simulink model "pro_simu_obsv"  (R2020b)
settings: Solver=VariableStepAuto  StartTime=0.0  StopTime=6  RelTol=1e-3
values from neighbouring files (symbols this model uses):
  A = subs(Jx,[x1,x2,x3,x4],[0,0,0,0])    [linearisation.m]    (also in pro_main_code.m = [0 1 0 0;0 -15.47 41.68 0;0 0 0 1;0 -14.89 84.05 0])
  B = subs(Ju,u,0)    [linearisation.m]    (also in pro_main_code.m = [0;27.12;0;23.13])
  C = [1 0 0 0]    [pro_main_code.m]
  Gcl0_inv_lqr = inv(Gcl0)    [pro_main_code.m]
  K_11_lqr = K_lqr1(1,1:4)    [pro_main_code.m]
  K_12_lqr = K_lqr1(1,5)    [pro_main_code.m]
  K_lqr = lqr(A,B,QQ,R)    [pro_main_code.m]
  L_lqr = l_lqr'    [pro_main_code.m]
libraries: simulink x1
settings Model: Creator=Benyamin (hamireZ)  LastModifiedBy=Benyamin (hamireZ)

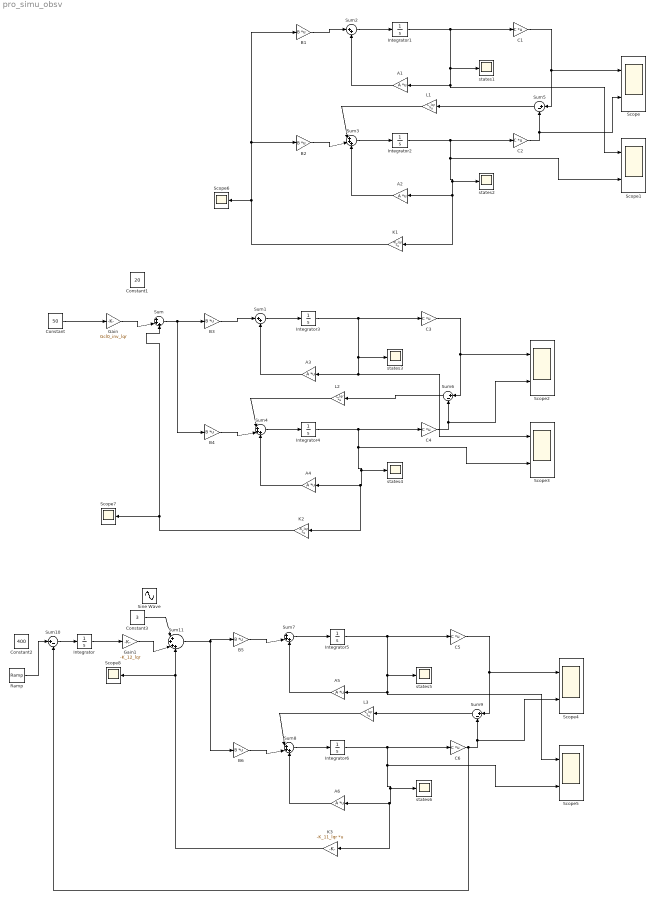
== system pro_simu_obsv ==
  A{1..6} (6 alike) : Gain  Gain=A  Multiplication=Matrix(K*u) (u vector)
  B{1..6} (6 alike) : Gain  Gain=B  Multiplication=Matrix(K*u) (u vector)
  C{1..6} (6 alike) : Gain  Gain=C  Multiplication=Matrix(K*u) (u vector)
  Constant : Constant  Value=50
  Constant1 : Constant  Value=20
  Constant2 : Constant  Value=400
  Constant3 : Constant  Value=3
  Gain : Gain  Gain=Gcl0_inv_lqr
  Gain1 : Gain  Gain=-K_12_lqr
  Integrator : Integrator
  Integrator1 : Integrator  InitialCondition=[1;0;1;0]
  Integrator2 : Integrator  InitialCondition=[-1;0;0;0]
  Integrator3 : Integrator  InitialCondition=[1;1;1;1]
  Integrator4 : Integrator  InitialCondition=[-1;0;-2;-1]
  Integrator5 : Integrator  InitialCondition=[1;1;1;1]
  Integrator6 : Integrator  InitialCondition=[-1;0;-2;-1]
  K1 : Gain  Gain=-K_lqr  Multiplication=Matrix(K*u) (u vector)
  K2 : Gain  Gain=-K_lqr  Multiplication=Matrix(K*u) (u vector)
  K3 : Gain  Gain=-K_11_lqr  Multiplication=Matrix(K*u) (u vector)
  L1 : Gain  Gain=L_lqr  Multiplication=Matrix(K*u) (u vector)
  L2 : Gain  Gain=L_lqr  Multiplication=Matrix(K*u) (u vector)
  L3 : Gain  Gain=L_lqr  Multiplication=Matrix(K*u) (u vector)
  Ramp : simulink/Sources/Ramp  slope=100  start=0  InitialOutput=0
  Scope{,1..5} (6 alike) : Scope  NumInputPorts=2
  Scope6 : Scope
  Scope7 : Scope
  Scope8 : Scope
  Sine Wave : Sin  Frequency=2  SampleTime=0
  Sum{,3..4,7..8} (5 alike) : Sum  Inputs=|+++
  Sum1 : Sum  Inputs=|++
  Sum{5..6,9..10} (4 alike) : Sum  Inputs=|+-
  Sum11 : Sum  Inputs=|++++
  Sum2 : Sum  Inputs=|++
  states{1..6} (6 alike) : Scope
  wires:
  Integrator6/1 -> C6/1, states6/1, A6/1, K3/1, Scope5/2
  B4/1 -> Sum4/2
  Sum1/1 -> Integrator3/1
  Constant/1 -> Gain/1
  Sum10/1 -> Integrator/1
  A3/1 -> Sum1/2
  C5/1 -> Scope4/1, Sum9/1
  Integrator/1 -> Gain1/1
  C4/1 -> Sum6/2, Scope2/2
  Gain1/1 -> Sum11/3
  Sum11/1 -> B5/1, B6/1
  B2/1 -> Sum3/2
  L1/1 -> Sum3/1
  Gain/1 -> Sum/2
  A4/1 -> Sum4/3
  Integrator5/1 -> A5/1, Scope5/1, states5/1, C5/1
  Sum6/1 -> L2/1
  Integrator3/1 -> A3/1, Scope3/1, states3/1, C3/1
  Sum4/1 -> Integrator4/1
  C3/1 -> Scope2/1, Sum6/1
  B5/1 -> Sum7/2
  B6/1 -> Sum8/2
  Integrator1/1 -> C1/1, states1/1, Scope1/1, A1/1
  C6/1 -> Sum9/2, Scope4/2, Sum10/2
  Sum8/1 -> Integrator6/1
  Sum9/1 -> L3/1
  A5/1 -> Sum7/3
  Sum5/1 -> L1/1
  Sum/1 -> B4/1, B3/1
  L3/1 -> Sum8/1
  C2/1 -> Scope/2, Sum5/2
  A6/1 -> Sum8/3
  Integrator4/1 -> C4/1, states4/1, A4/1, K2/1, Scope3/2
  K3/1 -> Scope8/1, Sum11/4
  K1/1 -> Scope6/1, B2/1, B1/1
  C1/1 -> Sum5/1, Scope/1
  Integrator2/1 -> Scope1/2, K1/1, A2/1, states2/1, C2/1
  Sum7/1 -> Integrator5/1
  A1/1 -> Sum2/2
  B3/1 -> Sum1/1
  L2/1 -> Sum4/1
  A2/1 -> Sum3/3
  B1/1 -> Sum2/1
  Sum3/1 -> Integrator2/1
  Sum2/1 -> Integrator1/1
  K2/1 -> Scope7/1, Sum/3
  Ramp/1 -> Sum10/1
  Constant3/1 -> Sum11/1
